simulink model "sixth_10_03_25class"  (R2024a)
settings: Solver=VariableStepAuto  StartTime=0.0  StopTime=10.0  MaxStep=1e-5  RelTol=1e-3
undefined symbols (not defined in the file): fsw, l, r
libraries: simulink x4
settings Model: Creator=claudio.rossi  LastModifiedBy=s0001205361
settings OptimizationCC: ReuseModelBlockBuffer=off
settings RTWCC: GPUComputeCapability=3.5

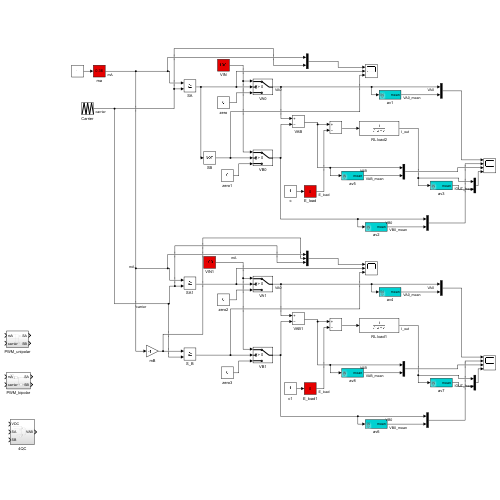
[thumbnail: Simulink's stored preview of the top-level diagram]
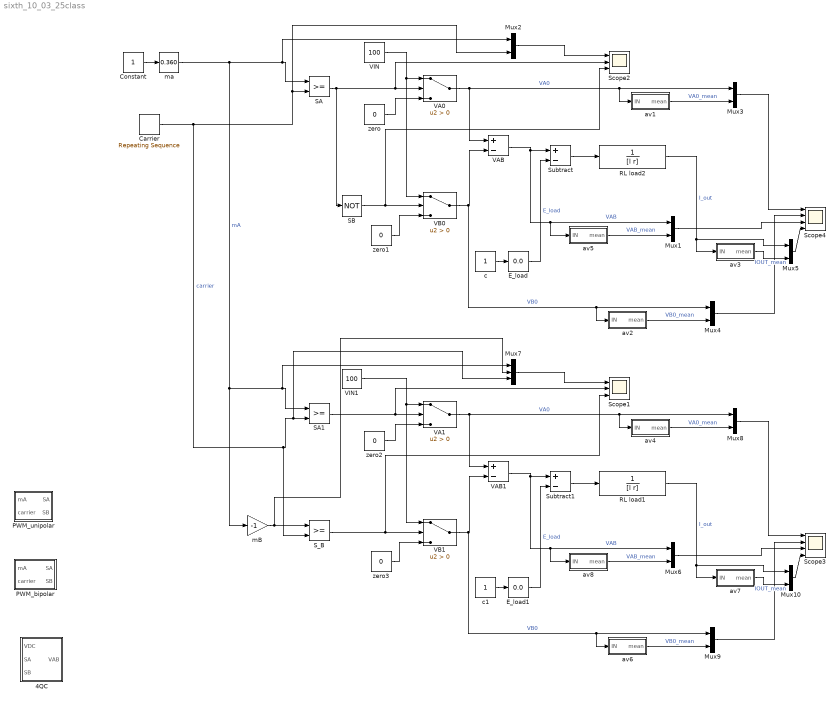
== system sixth_10_03_25class ==
  4QC : Subsystem
  "Carrier " : simulink/Sources/Repeating Sequence  rep_seq_t=[0 0.5/fsw 1/fsw]  rep_seq_y=[-1 1 -1 ]
  Constant : Constant
  E_load : simulink/Math Operations/Slider Gain  gain=0.0  low=0  high=200
  E_load1 : simulink/Math Operations/Slider Gain  gain=0.0  low=0  high=200
  Mux{1..6,8..10} (9 alike) : Mux  Inputs=2
  Mux7 : Mux  Inputs=3
  PWM_bipolar : Subsystem
  PWM_unipolar : Subsystem
  RL load1 : TransferFcn  Denominator=[l r]
  RL load2 : TransferFcn  Denominator=[l r]
  SA : RelationalOperator  OutDataTypeStr=boolean  RndMeth=Simplest  InputSameDT=off
  SA1 : RelationalOperator  OutDataTypeStr=boolean  RndMeth=Simplest  InputSameDT=off
  SB : Logic  Operator=NOT  AllPortsSameDT=off  OutDataTypeStr=boolean
  S_B : RelationalOperator  OutDataTypeStr=boolean  RndMeth=Simplest  InputSameDT=off
  Scope1 : Scope  NumInputPorts=3
  Scope2 : Scope  NumInputPorts=3
  Scope3 : Scope  NumInputPorts=4
  Scope4 : Scope  NumInputPorts=4
  Subtract : Sum  Inputs=+-
  Subtract1 : Sum  Inputs=+-
  VA0 : Switch  Criteria=u2 > Threshold  SaturateOnIntegerOverflow=off  InputSameDT=off
  VA1 : Switch  Criteria=u2 > Threshold  SaturateOnIntegerOverflow=off  InputSameDT=off
  VAB : Sum  Inputs=+-
  VAB1 : Sum  Inputs=+-
  VB0 : Switch  Criteria=u2 > Threshold  SaturateOnIntegerOverflow=off  InputSameDT=off
  VB1 : Switch  Criteria=u2 > Threshold  SaturateOnIntegerOverflow=off  InputSameDT=off
  VIN : Constant  Value=100
  VIN1 : Constant  Value=100
  av1 : Subsystem  mask{period=1/fsw}
      mask prompts: period "period [s]"
      mask DialogControl DescTextVar Prompt: calculate the averge over period
      mask DialogControl text Prompt: test
  av2 : Subsystem  mask{period=1/fsw}
      mask prompts: period "period [s]"
      mask DialogControl DescTextVar Prompt: calculate the averge over period
      mask DialogControl text Prompt: test
  av3 : Subsystem  mask{period=1/fsw}
      mask prompts: period "period [s]"
      mask DialogControl DescTextVar Prompt: calculate the averge over period
      mask DialogControl text Prompt: test
  av4 : Subsystem  mask{period=1/fsw}
      mask prompts: period "period [s]"
      mask DialogControl DescTextVar Prompt: calculate the averge over period
      mask DialogControl text Prompt: test
  av5 : Subsystem  mask{period=1/fsw}
      mask prompts: period "period [s]"
      mask DialogControl DescTextVar Prompt: calculate the averge over period
      mask DialogControl text Prompt: test
  av6 : Subsystem  mask{period=1/fsw}
      mask prompts: period "period [s]"
      mask DialogControl DescTextVar Prompt: calculate the averge over period
      mask DialogControl text Prompt: test
  av7 : Subsystem  mask{period=1/fsw}
      mask prompts: period "period [s]"
      mask DialogControl DescTextVar Prompt: calculate the averge over period
      mask DialogControl text Prompt: test
  av8 : Subsystem  mask{period=1/fsw}
      mask prompts: period "period [s]"
      mask DialogControl DescTextVar Prompt: calculate the averge over period
      mask DialogControl text Prompt: test
  c : Constant
  c1 : Constant
  mB : Gain  Gain=-1
  ma : simulink/Math Operations/Slider Gain  gain=0.360  low=-1  high=1
  zero{,1..3} (4 alike) : Constant  Value=0
  wires:
  ma/1 -> mB/1, SA1/1, Mux7/1, Mux2/1, SA/1  "mA"
  "Carrier "/1 -> S_B/2, Mux7/3, SA1/2, Mux2/2, SA/2  "carrier"
  Constant/1 -> ma/1
  SA/1 -> SB/1, Scope2/2, VA0/2
  zero/1 -> VA0/3
  zero1/1 -> VB0/3
  VIN/1 -> VB0/1, VA0/1
  SB/1 -> VB0/2, Scope2/3
  VA0/1 -> av1/1(IN), Mux3/1, VAB/1  "VA0"
  VAB/1 -> av5/1(IN), Mux1/1, Subtract/1  "VAB"
  c/1 -> E_load/1
  E_load/1 -> Subtract/2  "E_load"
  Subtract/1 -> RL load2/1
  Mux2/1 -> Scope2/1
  av5/1(mean) -> Mux1/2  "VAB_mean"
  Mux1/1 -> Scope4/3
  Mux3/1 -> Scope4/1
  av1/1(mean) -> Mux3/2  "VA0_mean"
  av2/1(mean) -> Mux4/2  "VB0_mean"
  VB0/1 -> av2/1(IN), Mux4/1, VAB/2  "VB0"
  Mux4/1 -> Scope4/2
  Mux5/1 -> Scope4/4
  av3/1(mean) -> Mux5/2  "IOUT_mean"
  RL load2/1 -> Mux5/1, av3/1(IN)  "I_out"
  RL load1/1 -> av7/1(IN), Mux10/1  "I_out"
  av7/1(mean) -> Mux10/2  "IOUT_mean"
  Mux10/1 -> Scope3/4
  Mux9/1 -> Scope3/2
  VB1/1 -> VAB1/2, Mux9/1, av6/1(IN)  "VB0"
  av6/1(mean) -> Mux9/2  "VB0_mean"
  av4/1(mean) -> Mux8/2  "VA0_mean"
  Mux8/1 -> Scope3/1
  Mux6/1 -> Scope3/3
  av8/1(mean) -> Mux6/2  "VAB_mean"
  Mux7/1 -> Scope1/1
  Subtract1/1 -> RL load1/1
  E_load1/1 -> Subtract1/2  "E_load"
  c1/1 -> E_load1/1
  VAB1/1 -> Subtract1/1, Mux6/1, av8/1(IN)  "VAB"
  VA1/1 -> VAB1/1, Mux8/1, av4/1(IN)  "VA0"
  S_B/1 -> Scope1/3, VB1/2
  VIN1/1 -> VA1/1, VB1/1
  zero3/1 -> VB1/3
  zero2/1 -> VA1/3
  SA1/1 -> VA1/2, Scope1/2
  mB/1 -> Mux7/2, S_B/1

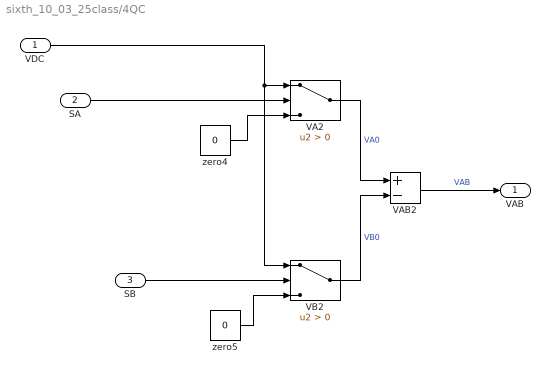
== system sixth_10_03_25class/4QC ==
  VDC : Inport
  SA : Inport  Port=2
  SB : Inport  Port=3
  VA2 : Switch  Criteria=u2 > Threshold  SaturateOnIntegerOverflow=off  InputSameDT=off
  VAB2 : Sum  Inputs=+-
  VB2 : Switch  Criteria=u2 > Threshold  SaturateOnIntegerOverflow=off  InputSameDT=off
  zero4 : Constant  Value=0
  zero5 : Constant  Value=0
  VAB : Outport
  wires:
  zero5/1 -> VB2/3
  SB/1 -> VB2/2
  zero4/1 -> VA2/3
  VDC/1 -> VA2/1, VB2/1
  SA/1 -> VA2/2
  VA2/1 -> VAB2/1  "VA0"
  VAB2/1 -> VAB/1  "VAB"
  VB2/1 -> VAB2/2  "VB0"

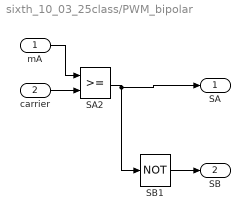
== system sixth_10_03_25class/PWM_bipolar ==
  mA : Inport
  carrier : Inport  Port=2
  SA2 : RelationalOperator  OutDataTypeStr=boolean  RndMeth=Simplest  InputSameDT=off
  SB1 : Logic  Operator=NOT  AllPortsSameDT=off  OutDataTypeStr=boolean
  SA : Outport
  SB : Outport  Port=2
  wires:
  SA2/1 -> SA/1, SB1/1
  mA/1 -> SA2/1
  carrier/1 -> SA2/2
  SB1/1 -> SB/1

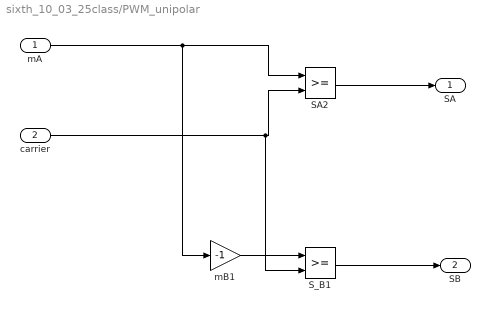
== system sixth_10_03_25class/PWM_unipolar ==
  mA : Inport
  carrier : Inport  Port=2
  SA2 : RelationalOperator  OutDataTypeStr=boolean  RndMeth=Simplest  InputSameDT=off
  S_B1 : RelationalOperator  OutDataTypeStr=boolean  RndMeth=Simplest  InputSameDT=off
  mB1 : Gain  Gain=-1
  SA : Outport
  SB : Outport  Port=2
  wires:
  mA/1 -> mB1/1, SA2/1
  carrier/1 -> S_B1/2, SA2/2
  SA2/1 -> SA/1
  mB1/1 -> S_B1/1
  S_B1/1 -> SB/1

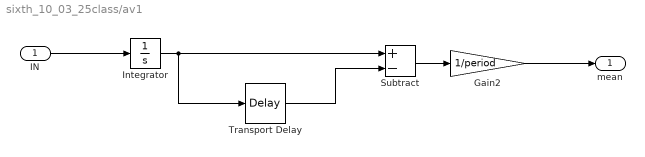
== system sixth_10_03_25class/av1 ==
  IN : Inport
  Gain2 : Gain  Gain=1/period
  Integrator : Integrator
  Subtract : Sum  Inputs=+-
  Transport Delay : TransportDelay  DelayTime=period
  mean : Outport
  wires:
  Integrator/1 -> Transport Delay/1, Subtract/1
  Gain2/1 -> mean/1
  Subtract/1 -> Gain2/1
  Transport Delay/1 -> Subtract/2
  IN/1 -> Integrator/1

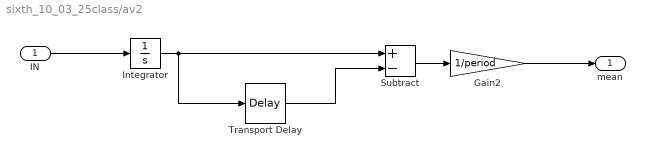
== system sixth_10_03_25class/av2 ==
  IN : Inport
  Gain2 : Gain  Gain=1/period
  Integrator : Integrator
  Subtract : Sum  Inputs=+-
  Transport Delay : TransportDelay  DelayTime=period
  mean : Outport
  wires:
  IN/1 -> Integrator/1
  Transport Delay/1 -> Subtract/2
  Subtract/1 -> Gain2/1
  Gain2/1 -> mean/1
  Integrator/1 -> Subtract/1, Transport Delay/1

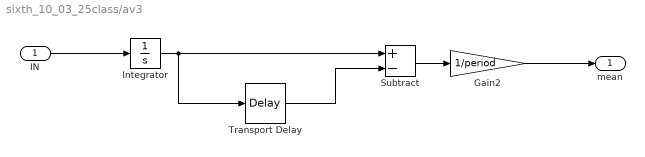
== system sixth_10_03_25class/av3 ==
  IN : Inport
  Gain2 : Gain  Gain=1/period
  Integrator : Integrator
  Subtract : Sum  Inputs=+-
  Transport Delay : TransportDelay  DelayTime=period
  mean : Outport
  wires:
  Integrator/1 -> Transport Delay/1, Subtract/1
  Gain2/1 -> mean/1
  Subtract/1 -> Gain2/1
  Transport Delay/1 -> Subtract/2
  IN/1 -> Integrator/1

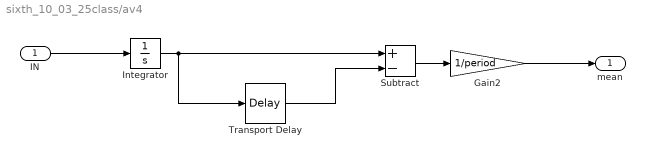
== system sixth_10_03_25class/av4 ==
  IN : Inport
  Gain2 : Gain  Gain=1/period
  Integrator : Integrator
  Subtract : Sum  Inputs=+-
  Transport Delay : TransportDelay  DelayTime=period
  mean : Outport
  wires:
  IN/1 -> Integrator/1
  Transport Delay/1 -> Subtract/2
  Subtract/1 -> Gain2/1
  Gain2/1 -> mean/1
  Integrator/1 -> Subtract/1, Transport Delay/1

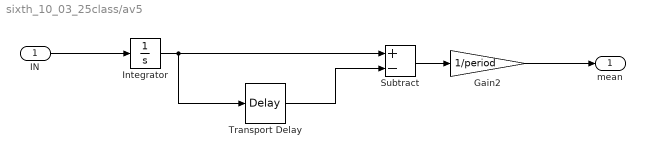
== system sixth_10_03_25class/av5 ==
  IN : Inport
  Gain2 : Gain  Gain=1/period
  Integrator : Integrator
  Subtract : Sum  Inputs=+-
  Transport Delay : TransportDelay  DelayTime=period
  mean : Outport
  wires:
  IN/1 -> Integrator/1
  Transport Delay/1 -> Subtract/2
  Subtract/1 -> Gain2/1
  Gain2/1 -> mean/1
  Integrator/1 -> Subtract/1, Transport Delay/1

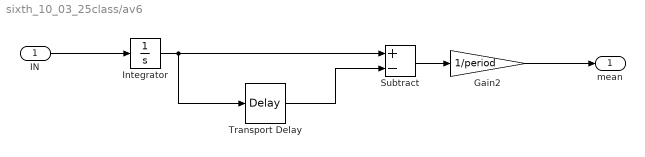
== system sixth_10_03_25class/av6 ==
  IN : Inport
  Gain2 : Gain  Gain=1/period
  Integrator : Integrator
  Subtract : Sum  Inputs=+-
  Transport Delay : TransportDelay  DelayTime=period
  mean : Outport
  wires:
  Integrator/1 -> Transport Delay/1, Subtract/1
  Gain2/1 -> mean/1
  Subtract/1 -> Gain2/1
  Transport Delay/1 -> Subtract/2
  IN/1 -> Integrator/1

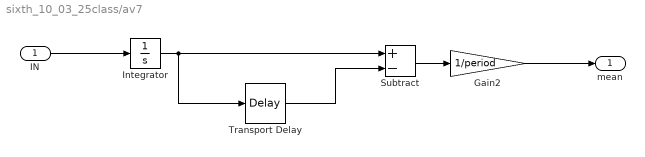
== system sixth_10_03_25class/av7 ==
  IN : Inport
  Gain2 : Gain  Gain=1/period
  Integrator : Integrator
  Subtract : Sum  Inputs=+-
  Transport Delay : TransportDelay  DelayTime=period
  mean : Outport
  wires:
  IN/1 -> Integrator/1
  Transport Delay/1 -> Subtract/2
  Subtract/1 -> Gain2/1
  Gain2/1 -> mean/1
  Integrator/1 -> Subtract/1, Transport Delay/1

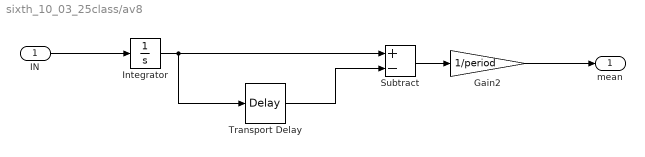
== system sixth_10_03_25class/av8 ==
  IN : Inport
  Gain2 : Gain  Gain=1/period
  Integrator : Integrator
  Subtract : Sum  Inputs=+-
  Transport Delay : TransportDelay  DelayTime=period
  mean : Outport
  wires:
  Integrator/1 -> Transport Delay/1, Subtract/1
  Gain2/1 -> mean/1
  Subtract/1 -> Gain2/1
  Transport Delay/1 -> Subtract/2
  IN/1 -> Integrator/1
